simulink model "pendulumWithDampingAndFeedback"  (Simulink 7.2)
settings: Solver=ode45  StartTime=0.0  StopTime=100.0  RelTol=1e-3
undefined symbols (not defined in the file or in its folder): d, g, L, m
libraries: simulink x2
settings Model: Creator=mauricio  LastModifiedBy=mauricio
settings DebuggingCC: SolverPrmCheckMsg=none

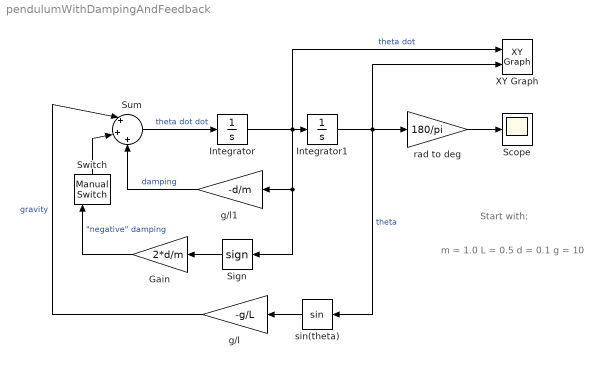
== system pendulumWithDampingAndFeedback ==
  note: Start with:
  note: m = 1.0
      | L = 0.5
      |  d = 0.1
      | g = 10
  Gain : Gain  Orientation=left  Gain=2*d/m  ParameterDataType=sfix(16)  ParameterScaling=2^0  OutDataType=sfix(16)  OutScaling=2^0
  Integrator : Integrator
  Integrator1 : Integrator  InitialCondition=pi/6
  Scope : Scope
      settings: YMin=-45  YMax=45
  Sign : Signum  Orientation=left
  Sum : Sum  Inputs=|+|+|+  OutDataType=sfix(16)  OutScaling=2^0
  Switch : simulink/Signal Routing/Manual Switch  Orientation=up  SystemSampleTime=-1  sw=1  action=0  varsize=off
  XY Graph : simulink/Sinks/XY Graph  SystemSampleTime=-1  xmin=-3  xmax=3  ymin=-1  ymax=1  st=-1
  g/l : Gain  Orientation=left  Gain=-g/L  ParameterDataType=sfix(16)  ParameterScaling=2^0  OutDataType=sfix(16)  OutScaling=2^0
  g/l1 : Gain  Orientation=left  Gain=-d/m  ParameterDataType=sfix(16)  ParameterScaling=2^0  OutDataType=sfix(16)  OutScaling=2^0
  rad to deg : Gain  Gain=180/pi  ParameterDataType=sfix(16)  ParameterScaling=2^0  OutDataType=sfix(16)  OutScaling=2^0
  sin(theta) : Trigonometry  Orientation=left
  wires:
  Integrator/1 -> g/l1/1, Sign/1, Integrator1/1, XY Graph/1  "theta dot"
  Integrator1/1 -> rad to deg/1, sin(theta)/1, XY Graph/2  "theta"
  sin(theta)/1 -> g/l/1
  rad to deg/1 -> Scope/1
  Sum/1 -> Integrator/1  "theta dot dot"
  g/l/1 -> Sum/1  "gravity"
  g/l1/1 -> Sum/3  "damping"
  Gain/1 -> Switch/1  "\"negative\" damping"
  Sign/1 -> Gain/1
  Switch/1 -> Sum/2
